simulink model "ex13slidingattitude"  (R2025b)
settings: Solver=VariableStepAuto  StartTime=0.0  StopTime=250  RelTol=1e-3
values from neighbouring files (symbols this model uses):
  IJ = inv(J)    [ex13.m]    (also in ex6.m)
  J = jacobian(f,[x1,x2])    [ex1.m]    (also in ex13.m = diag([10400, 8200, 9200]); ex2.m; ex6.m = diag([7000,5900,9600]))
  q0 = [0.68438, -0.56827,-0.10002,-0.44574]'    [ex13.m]    (also in ex6.m = [1;0;0;0])
  w0 = [0;0;0]    [ex13.m]    (also in ex6.m)
  wr = [1;0;0]    [ex13.m]
libraries: vrlib x1
settings Model: Creator=Esteban  LastModifiedBy=Esteban

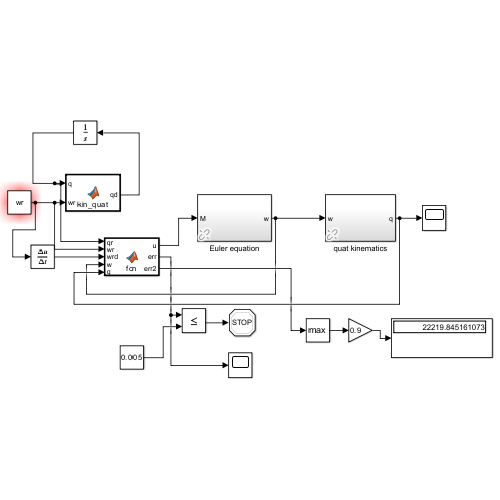
[thumbnail: Simulink's stored preview of the top-level diagram]
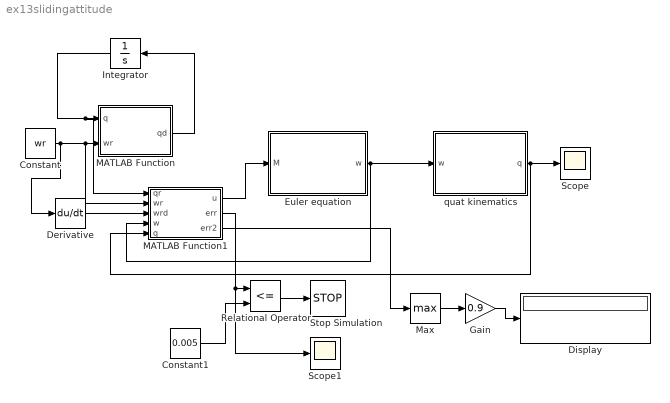
== system ex13slidingattitude ==
  Constant : Constant  Value=wr
  Constant1 : Constant  Value=0.005
  Derivative : Derivative
  Display : Display
      settings: Format=decimal (Stored Integer)
  Euler equation : Subsystem  AncestorBlock=lib_rotations_2014/Euler equation
  Gain : Gain  Gain=0.9
  Integrator : Integrator  InitialCondition=[1;0;0;0]
  MATLAB Function : MATLAB Function  TreatAsAtomicUnit=on
  MATLAB Function1 : MATLAB Function  TreatAsAtomicUnit=on
  Max : MinMax  Function=max
  Relational Operator : RelationalOperator  Operator=<=  OutDataTypeStr=boolean  RndMeth=Simplest  InputSameDT=off
  Scope : Scope
  Scope1 : Scope
      settings: ActiveDisplayYMinimum=-1  ActiveDisplayYMaximum=1
  Stop Simulation : Stop
  quat kinematics : Subsystem  AncestorBlock=lib_rotations_2014/quat kinematics
  wires:
  Constant/1 -> Derivative/1, MATLAB Function1/2(wr), MATLAB Function/2(wr)
  MATLAB Function/1(qd) -> Integrator/1
  Integrator/1 -> MATLAB Function1/1(qr), MATLAB Function/1(q)
  Derivative/1 -> MATLAB Function1/3(wrd)
  MATLAB Function1/1(u) -> Euler equation/1(M)
  Euler equation/1(w) -> MATLAB Function1/4(w), quat kinematics/1(w)
  quat kinematics/1(q) -> MATLAB Function1/5(q), Scope/1
  Constant1/1 -> Relational Operator/2
  MATLAB Function1/2(err) -> Scope1/1, Relational Operator/1
  Relational Operator/1 -> Stop Simulation/1
  MATLAB Function1/3(err2) -> Max/1
  Max/1 -> Gain/1
  Gain/1 -> Display/1

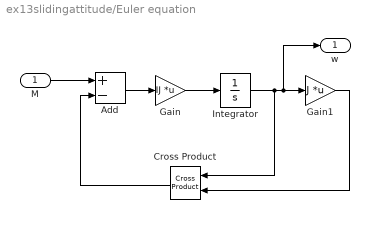
== system ex13slidingattitude/Euler equation ==
  M : Inport
  Add : Sum  Inputs=+-
  Cross Product : vrlib/Utilities/Cross Product
  Gain : Gain  Gain=IJ  Multiplication=Matrix(K*u)
  Gain1 : Gain  Gain=J  Multiplication=Matrix(K*u)
  Integrator : Integrator  InitialCondition=w0
  w : Outport  VectorParamsAs1DForOutWhenUnconnected=off
  wires:
  Cross Product/1 -> Add/2
  Add/1 -> Gain/1
  Gain1/1 -> Cross Product/2
  Gain/1 -> Integrator/1
  Integrator/1 -> Gain1/1, w/1, Cross Product/1
  M/1 -> Add/1

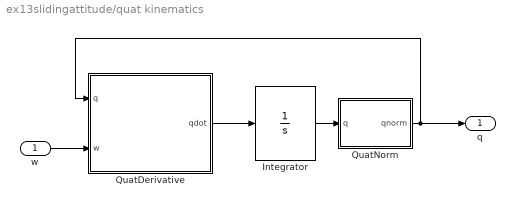
== system ex13slidingattitude/quat kinematics ==
  w : Inport  PortDimensions=3
  Integrator : Integrator  InitialCondition=q0
  QuatDerivative : MATLAB Function  TreatAsAtomicUnit=on
  QuatNorm : MATLAB Function  TreatAsAtomicUnit=on
  q : Outport  PortDimensions=4  VectorParamsAs1DForOutWhenUnconnected=off
  wires:
  w/1 -> QuatDerivative/2(w)
  QuatDerivative/1(qdot) -> Integrator/1
  QuatNorm/1(qnorm) -> QuatDerivative/1(q), q/1
  Integrator/1 -> QuatNorm/1(q)

== matlab function ex13slidingattitude/quat kinematics/QuatDerivative ==
  data: q input; qdot output; w input
function qdot= QuatDerivative(q,w)
%#codegen
omegaq=[0; w];
Q=[q(1) -q(2) -q(3) -q(4);
    q(2) q(1) -q(4) q(3);
    q(3) q(4) q(1) -q(2);
    q(4) -q(3) q(2) q(1)];
qdot=Q*omegaq/2;

== matlab function ex13slidingattitude/quat kinematics/QuatNorm ==
  data: q input; qnorm output
function qnorm = QuatNorm(q)
%#codegen
qnorm=zeros(4,1);
q2=sqrt(q'*q);
qnorm=q/q2;

== matlab function ex13slidingattitude/MATLAB Function ==
  data: q input; wr input; qd output
function qd=kin_quat(q,wr)

% w=[0.2*sin(t);
%     0.5*sin(2*t);
%     0];

q=q/norm(q);

Q=[-q(2) -q(3) -q(4)
    q(1) -q(4) q(3)
    q(4) q(1)  -q(2)
    -q(3) q(2) q(1)];

qd=1/2*Q*wr;

== matlab function ex13slidingattitude/MATLAB Function1 ==
  data: qr input; u output; wr input; wrd input; w input; q input; err output; err2 output
function [u,err,err2] = fcn(qr,wr,wrd,w,q)


k1 = 89.4337;
k2 =0.89474;
n = 178.9474;

J = diag([10400, 8200, 9200]);

qs = [q(1);-q(2:4)];
dq = quatprod(qs,qr);
err = norm(dq(2:4));

dw = wr-w;

us = J*(wrd+(k2/2)*(dq(1)*dw + cross(dq(2:4),wr+w))) + cross(w,J*w);

s = dw + k2*sign(dq(1))*dq(2:4);

u = us + k1*J*tanh(n*s);

err2 = norm(u);
